simulink model "ME419_Ex1_8"  (R2023b)
settings: Solver=VariableStepAuto  StartTime=0.0  StopTime=10.0  RelTol=1e-3
settings Model: Creator=aliawolken  LastModifiedBy=aliawolken

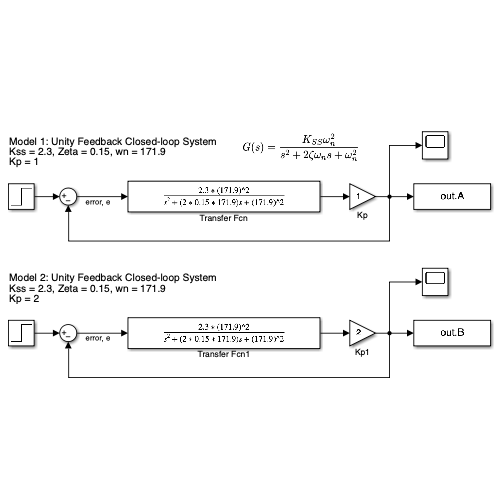
[thumbnail: Simulink's stored preview of the top-level diagram]
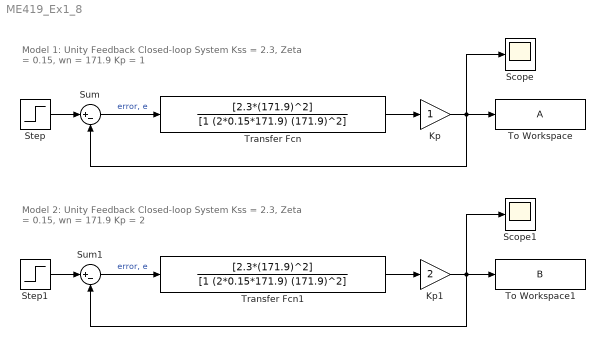
== system ME419_Ex1_8 ==
  note: Model 1: Unity Feedback Closed-loop System Kss = 2.3, Zeta = 0.15, wn = 171.9
      | Kp = 1
  note: Model 2: Unity Feedback Closed-loop System Kss = 2.3, Zeta = 0.15, wn = 171.9
      | Kp = 2
  Kp : Gain
  Kp1 : Gain  Gain=2
  Scope : Scope
  Scope1 : Scope
  Step : Step  SampleTime=0
  Step1 : Step  SampleTime=0
  Sum : Sum  Inputs=|+-
  Sum1 : Sum  Inputs=|+-
  To Workspace : ToWorkspace  VariableName=A  SampleTime=-1
  To Workspace1 : ToWorkspace  VariableName=B  SampleTime=-1
  Transfer Fcn : TransferFcn  Numerator=[2.3*(171.9)^2]  Denominator=[1 (2*0.15*171.9) (171.9)^2]
  Transfer Fcn1 : TransferFcn  Numerator=[2.3*(171.9)^2]  Denominator=[1 (2*0.15*171.9) (171.9)^2]
  wires:
  Transfer Fcn/1 -> Kp/1
  Sum/1 -> Transfer Fcn/1  "error, e"
  Step/1 -> Sum/1
  Kp/1 -> Scope/1, Sum/2, To Workspace/1
  Sum1/1 -> Transfer Fcn1/1  "error, e"
  Step1/1 -> Sum1/1
  Kp1/1 -> Scope1/1, Sum1/2, To Workspace1/1
  Transfer Fcn1/1 -> Kp1/1
